simulink library "db_pino_crem"  (R2018a)
settings: Solver=VariableStepAuto  StartTime=0.0  StopTime=10.0  RelTol=1e-3
undefined symbols (not defined in the file): B1, B2, J, K, M, R
settings Model: Creator=carma  LastModifiedBy=carma

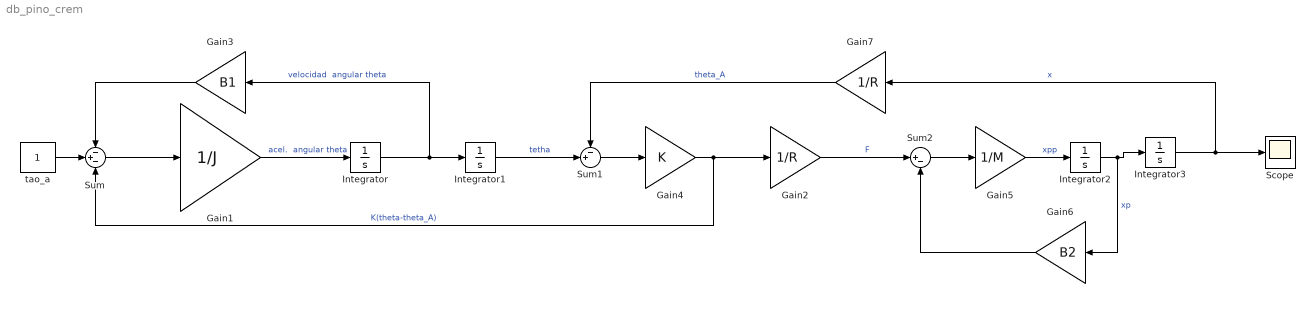
== system db_pino_crem ==
  Gain1 : Gain  Gain=1/J
  Gain2 : Gain  Gain=1/R
  Gain3 : Gain  Gain=B1
  Gain4 : Gain  Gain=K
  Gain5 : Gain  Gain=1/M
  Gain6 : Gain  Gain=B2
  Gain7 : Gain  Gain=1/R
  Integrator{,1..3} (4 alike) : Integrator
  Scope : Scope
  Sum : Sum  Inputs=-+-
  Sum1 : Sum  Inputs=-+|
  Sum2 : Sum  Inputs=|+-
  tao_a : Constant
  wires:
  Sum/1 -> Gain1/1
  Gain1/1 -> Integrator/1  "acel.  angular theta"
  Integrator/1 -> Gain3/1, Integrator1/1  "velocidad  angular theta"
  tao_a/1 -> Sum/2
  Gain3/1 -> Sum/1
  Sum1/1 -> Gain4/1
  Gain4/1 -> Sum/3, Gain2/1  "K(theta-theta_A)"
  Gain2/1 -> Sum2/1  "F"
  Integrator1/1 -> Sum1/2  "tetha"
  Gain7/1 -> Sum1/1  "theta_A"
  Sum2/1 -> Gain5/1
  Gain5/1 -> Integrator2/1  "xpp"
  Integrator2/1 -> Gain6/1, Integrator3/1  "xp"
  Integrator3/1 -> Gain7/1, Scope/1  "x"
  Gain6/1 -> Sum2/2
